simulink model "MATLABPSB_BASED_MODELING_AND_Sim"  (Simulink 8.1)
settings: Solver=FixedStepDiscrete  SolverMode=SingleTasking  StartTime=0.0  StopTime=1  FixedStep=Ts  MaxStep=Ts*2  RelTol=1e-4  AbsTol=1e-4
PreLoadFcn:
  | Ts=50e-6;
values from neighbouring files (symbols this model uses):
  A = 1.5    [LoadSimulation.m]
undefined symbols (not defined in the file or in its folder): DiscIntNeverNeededParam, find_system
libraries: powerlib x205, powerlib_extras x39
(part 1 of 5)
Description:
  | Copyright 2008-2012 The MathWorks, Inc.
settings Model: Creator=MathWorks  LastModifiedBy=LALIT  ExtModeTrigMode=oneshot  ExtModeArmWhenConnect=off  ExtModeAutoUpdateStatusClock=off
settings DataIOCC: LimitDataPoints=off  SaveFinalState=on  SaveFormat=StructureWithTime  SaveOutput=off  SaveTime=off  SignalLoggingName=sigsOut
settings OptimizationCC: BooleanDataType=off  InitFltsAndDblsToZero=on  EfficientMapNaN2IntZero=off
settings DebuggingCC: CheckExecutionContextPreStartOutputMsg=on  CheckExecutionContextRuntimeOutputMsg=on  SignalResolutionControl=TryResolveAllWithWarning  SolverPrmCheckMsg=none  MultiTaskDSMMsg=warning  MultiTaskCondExecSysMsg=none  StrictBusMsg=None
settings HardwareCC: TargetUnknown=on
settings RTWCC: IncludeERTFirstTime=on

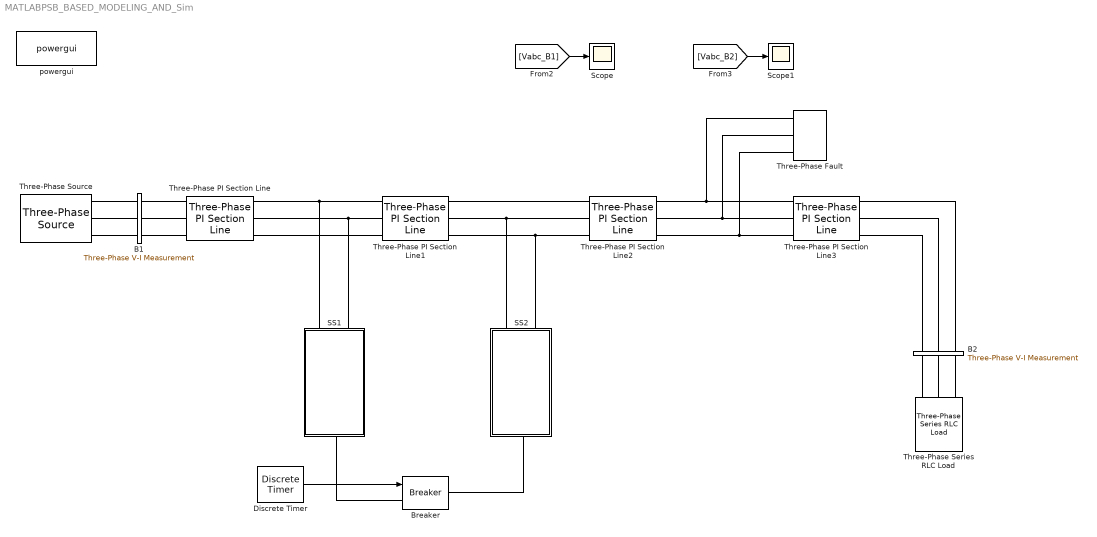
== system MATLABPSB_BASED_MODELING_AND_Sim ==
  B1 : powerlib/Measurements/Three-Phase V-I Measurement  VoltageMeasurement=phase-to-ground  SetLabelV=on  LabelV=Vabc_B1  Vpu=on  VpuLL=off  CurrentMeasurement=yes  SetLabelI=on  LabelI=Iabc_B1  Ipu=off  Pbase=100e6  Vbase=220e3  OutputType=Complex  PhasorSimulation=off  PSBequivalent=0
  B2 : powerlib/Measurements/Three-Phase V-I Measurement  VoltageMeasurement=phase-to-phase  SetLabelV=on  LabelV=Vabc_B2  Vpu=off  VpuLL=on  CurrentMeasurement=yes  SetLabelI=on  LabelI=Iabc_B2  Ipu=off  Pbase=100e6  Vbase=220e3  OutputType=Complex  PhasorSimulation=off  PSBequivalent=0
  Breaker : powerlib/Elements/Breaker  BreakerResistance=0.01  InitialState=0  SnubberResistance=1e6  SnubberCapacitance=inf  SwitchingTimes="[ 1/60  5/60 ]"  External=on  Measurements=None  MoreParameters=off  NoBreakLoop=off
  Discrete Timer : powerlib_extras/Discrete  Control Blocks/Discrete Timer  t=[0 1]  e=[0 1]  Ts=Ts
  SS1 : Subsystem
  SS2 : Subsystem
  Scope : Scope
      settings: SaveName=ScopeData10  Decimation=5
  Scope1 : Scope
      settings: YMin=-1.1  YMax=1.1  Decimation=5
  Three-Phase PI Section Line{,1..3} (4 alike) : powerlib/Elements/Three-Phase PI Section Line  LConnTagsString=a|b|c  RConnTagsString=A|B|C  Frequency=50  Resistances=[ 0.01273 0.3864]  Inductances="[ 0.9337e-3  4.1264e-3]"  Capacitances=[12.74e-9 7.751e-9]  Length=100
  Three-Phase Series RLC Load : powerlib/Elements/Three-Phase Series RLC Load  LConnTagsString=A|B|C  Configuration=Y (grounded)  NominalVoltage=220e3  NominalFrequency=50  ActivePower=100e6  InductivePower=0  CapacitivePower=0  Measurements=None  LoadType=constant Z
  Three-Phase Fault : powerlib/Elements/Three-Phase Fault  FaultA=on  FaultB=on  FaultC=on  FaultResistance=50  GroundFault=on  GroundResistance=0.001  External=off  SwitchStatus=[1]  SwitchTimes=[0.3]  InitialStates=[0 0 1]  SnubberResistance=1e6  SnubberCapacitance=inf  Measurements=None
  Three-Phase Source : powerlib/Electrical Sources/Three-Phase Source  Voltage=220e3  PhaseAngle=0  Frequency=50  InternalConnection=Yg  SpecifyImpedance=on  Resistance=0.8929  Inductance=16.58e-3  ShortCircuitLevel=5000e6  BaseVoltage=220e3  XRratio=7  BusType=swing  Pref=0  Qref=0  Qmin=-inf  Qmax=inf
  powergui : powerlib/powergui  Priority=2  SimulationMode=Discrete  SolverType=Tustin  SampleTime=Ts  frequency=60  SPID=off  DisableSnubberDevices=off  DisableRonSwitches=off  DisableVfSwitches=off  SwTol=0  Interpol=off  DisplayEquations=off  frequencyindice=50  Pbase=100e6  ErrMax=1e-4  Iterations=50  UnitsV=kV  UnitsW=MW  FunctionMessages=off  echomessages=off  HookPort=off  EnableUseOfTLC=off  x0status=blocks  RestoreLinks=warning  ResistiveCurrentMeasurement=off  Frange=[0:2:500]  Ylog=off  Xlog=on  ShowGrid=off  save=off  variable=ZData  structure=Va  ZoomFFT=off  StartTime=0.7  cycles=1  DisplayStyle=1  fundamental=60  FreqAxis=off  MaxFrequency=1000  frequencyindicesteady=1  RmsSteady=2  display=off  Ts=0  methode=off
  wires:
  [Vabc_B1] -> Scope/1
  [Vabc_B2] -> Scope1/1
  Discrete Timer/1 -> Breaker/1
  connections:
  SS1/LConn1 -- Three-Phase PI Section Line/RConn1 -- Three-Phase PI Section Line1/LConn1
  Three-Phase Fault/LConn1 -- Three-Phase PI Section Line2/RConn1 -- Three-Phase PI Section Line3/LConn1
  SS1/LConn2 -- Three-Phase PI Section Line/RConn2 -- Three-Phase PI Section Line1/LConn2
  Three-Phase PI Section Line2/LConn2 -- SS2/LConn1 -- Three-Phase PI Section Line1/RConn2
  Three-Phase PI Section Line2/LConn3 -- SS2/LConn2 -- Three-Phase PI Section Line1/RConn3
  Three-Phase Fault/LConn2 -- Three-Phase PI Section Line2/RConn2 -- Three-Phase PI Section Line3/LConn2
  Three-Phase Fault/LConn3 -- Three-Phase PI Section Line2/RConn3 -- Three-Phase PI Section Line3/LConn3
  Three-Phase Source/RConn1 -- B1/LConn1
  Three-Phase PI Section Line1/RConn1 -- Three-Phase PI Section Line2/LConn1
  B1/RConn3 -- Three-Phase PI Section Line/LConn3
  Three-Phase Source/RConn3 -- B1/LConn3
  Three-Phase PI Section Line3/RConn1 -- B2/LConn3
  Three-Phase Source/RConn2 -- B1/LConn2
  B1/RConn1 -- Three-Phase PI Section Line/LConn1
  B1/RConn2 -- Three-Phase PI Section Line/LConn2
  B2/RConn1 -- Three-Phase Series RLC Load/LConn1
  Breaker/LConn1 -- SS1/RConn1
  Breaker/RConn1 -- SS2/RConn1
  B2/RConn2 -- Three-Phase Series RLC Load/LConn2
  Three-Phase PI Section Line3/RConn3 -- B2/LConn1
  Three-Phase PI Section Line/RConn3 -- Three-Phase PI Section Line1/LConn3
  Three-Phase PI Section Line3/RConn2 -- B2/LConn2
  B2/RConn3 -- Three-Phase Series RLC Load/LConn3

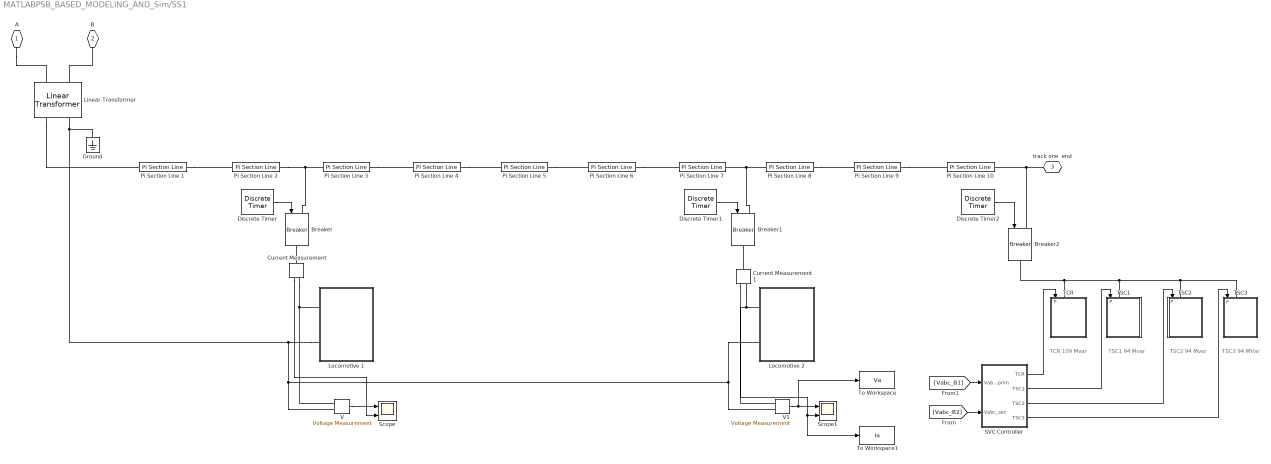
== system MATLABPSB_BASED_MODELING_AND_Sim/SS1 ==
  note: TSC1
      | 94 Mvar
  note: TCR
      | 109 Mvar
  note: TSC2
      | 94 Mvar
  note: TSC3
      | 94 MVar
  Breaker : powerlib/Elements/Breaker  BreakerResistance=0.01  InitialState=0  SnubberResistance=1e6  SnubberCapacitance=inf  SwitchingTimes="[ 1/60  5/60 ]"  External=on  Measurements=None  MoreParameters=off  NoBreakLoop=off
  Breaker1 : powerlib/Elements/Breaker  BreakerResistance=0.01  InitialState=0  SnubberResistance=1e6  SnubberCapacitance=inf  SwitchingTimes="[ 1/60  5/60 ]"  External=on  Measurements=None  MoreParameters=off  NoBreakLoop=off
  Breaker2 : powerlib/Elements/Breaker  BreakerResistance=0.01  InitialState=0  SnubberResistance=1e6  SnubberCapacitance=inf  SwitchingTimes="[ 1/60  5/60 ]"  External=on  Measurements=None  MoreParameters=off  NoBreakLoop=off
  Current Measurement : powerlib/Measurements/Current Measurement  PhasorSimulation=off  OutputType=Complex  PSBequivalent=0
  Current Measurement1 : powerlib/Measurements/Current Measurement  PhasorSimulation=off  OutputType=Complex  PSBequivalent=0
  Discrete Timer : powerlib_extras/Discrete  Control Blocks/Discrete Timer  t=[0 0.01]  e=[0 1]  Ts=Ts
  Discrete Timer1 : powerlib_extras/Discrete  Control Blocks/Discrete Timer  t=[0 0.1]  e=[0 1]  Ts=Ts
  Discrete Timer2 : powerlib_extras/Discrete  Control Blocks/Discrete Timer  t=[0 0.6]  e=[0 1]  Ts=Ts
  Ground : powerlib/Elements/Ground  LConnTagsString=a
  Linear Transformer : powerlib/Elements/Linear Transformer  LConnTagsString=a|b  RConnTagsString=A|B  UNITS=pu  NominalPower=[ 25e6 50 ]  winding1="[ 220e3  0.001  0.06 ]"  winding2="[ 25e3  0.001  0.06 ]"  ThreeWindings=off  winding3=[ 315e3 0.002 0.08 ]  RmLm=[ 500 500 ]  Measurements=None  DataType=off
  Locomotive 1 : Subsystem
  Locomotive 2 : Subsystem
  Pi Section Line {1..10} (10 alike) : powerlib/Elements/Pi Section Line  LConnTagsString=__new0  RConnTagsString=__new0  Frequency=50  Resistance=0.169  Inductance=0.432/(2*pi*50)  Capacitance=0.011e-6  Length=4  PiSections=1  Measurements=None
      settings: AttributesFormatString=\n
  SVC Controller : Subsystem  mask(SVC Controller){OpMode=Voltage regulation, Vref=1.0, KpKi=[0 800], Xs=0.01, Bmin_max=[-1.04  3.23], Bref=0, Ts=Ts}
      mask prompts: OpMode "Operation mode"; Vref "Reference voltage (pu):"; KpKi "Regulator gains [ Kp  Ki ]:"; Xs "Droop (pu/100MVA):"; Bmin_max "Min. and max. primary susceptances [ Bind Bcap] (pu/100MVA):"; Bref "Susceptance Bref (pu/100MVA) (Var control mode):"; Ts "Sample time (s):"
      mask help:
      | This block implements a controller for a Static Var Compensator (SVC) consisting of one thyristor-controlled reactor bank (TCR) and three thyristor-switched capacitor banks (TSCs). Outputs TCR, TSC1, TSC2 and TSC3 are vectors of six pulses for the TCR and the three TSCs.
      | In Voltage control mode the primary voltage (Vabc_prim) is controlled at Vref within the maximum inductive and capacitive susceptance range and droop setting. In Var control mode the SVC susceptance  is  kept constant at Bref (Bref<0 for inductive mode).
      | Thyristor pulses are synchronized on secondary line-to-line voltages (Vabc_sec) of the coupling transformer, assuming a Wye/Delta (D1) connection.
      mask init:
      | Kp=KpKi(1);
      | Ki=KpKi(2);
      | Bmin=Bmin_max(1);
      | Bmax=Bmin_max(2);
      mask TypeOptions OpMode: Voltage regulation | Var control (Fixed susceptance Bref)
  Scope : Scope  NumInputPorts=2
      settings: YMin=-40000~-5  YMax=40000~5  SaveName=ScopeData8  Decimation=5
  Scope1 : Scope  NumInputPorts=2
      settings: YMin=-40000~-5  YMax=40000~5  SaveName=ScopeData9  Decimation=5
  TCR : Subsystem  LoadFcn=find_system(gcs,'FollowLinks', 'on', 'LookUnderMasks', 'all');  mask(TCR branch){Ltcr=18.7e-3, Q=50, ParS=[500 250e-9], ParT=[1e-3  1*15]}
      mask prompts: Ltcr "TCR Inductance (H) :"; Q "Quality factor:"; ParS "Thyristor snubber: [ R (ohm)   C (F)  ]"; ParT "Thyristor data: [ Ron (ohm)   Vf (volt) ]"
      mask init:
      | Rtcr=(2*pi*60) * Ltcr / Q;
      | Rsnub=ParS(1);
      | Csnub=ParS(2);
      | Ron=ParT(1);
      | Vf=ParT(2);
      mask Display:
      | plot(0,0);plot(125,220)
      | plot([62 62 37 37 49 25 37],[15 39 39 58 76 76 58])
      | plot([62 87 87 99 87 75 87],[39 39 58 58 76 58 58])
      | plot([25 49],[58 58]);plot([37 25],[58 49])
      | plot([75 99],[76 76]);plot([87 99],[76 85])
      | plot([37 37 87 87],[76 95 95 76])
      | plot([62 62],[95 122]);plot([62 62],[164 186])
      | plot([62 72 78 79 78 72 62],[122 123 125 129 133 135 136])
      | plot([62 72 78 79 78 72 62],14+[122 123 125 129 133 135 136])
      | plot([62 72 78 79 78 72 62],28+[122 123 125 129 133 135 136])
  TSC1 : Subsystem  mask(TSC branch){Ccmt=308.4e-6, ParL=[1.13e-3 4.26e-3*2 191.7/2], ParS=[500 250e-9], ParT=[1e-3  1*15]}
      mask prompts: Ccmt "Capacitance (F) :"; ParL "[ Inductance (H)  Rseries (ohm)  Rparallel (ohm)  ]"; ParS "Thyristor snubber: [ R (ohm)   C (F)  ]"; ParT "Thyristor data: [ Ron (ohm)  Vf (volt) ]"
      mask init:
      | Lcmt=ParL(1);
      | Rseries=ParL(2);
      | Rparallel=ParL(3);
      | Rsnub=ParS(1);
      | Csnub=ParS(2);
      | Ron=ParT(1);
      | Vf=ParT(2);
      mask Display:
      | plot(0,0);plot(125,220)
      | plot([62 62 37 37 49 25 37],[15 39 39 58 76 76 58])
      | plot([62 87 87 99 87 75 87],[39 39 58 58 76 58 58])
      | plot([25 49],[58 58]);plot([37 25],[58 49])
      | plot([75 99],[76 76]);plot([87 99],[76 85])
      | plot([37 37 87 87],[76 95 95 76])
      | plot([62 62],[95 133]);plot([62 62],[164 183])
      | plot([62 69 73 78 81 82],13+[120 120 119 118 117 115])
      | plot([62 55 51 46 43 42],13+[120 120 119 118 117 115])
      | plot([42 82],[145 145])
      | plot([62 62],[145 164])
  TSC2 : Subsystem  mask(TSC branch){Ccmt=308.4e-6, ParL=[1.13e-3 4.26e-3*2 191.7/2], ParS=[500 250e-9], ParT=[1e-3 1*15]}
      mask prompts: Ccmt "Capacitance (F) :"; ParL "[ Inductance (H)  Rseries (ohm)  Rparallel (ohm)  ]"; ParS "Thyristor snubber: [ R (ohm)   C (F)  ]"; ParT "Thyristor data: [ Ron (ohm)  Vf (volt) ]"
      mask init:
      | Lcmt=ParL(1);
      | Rseries=ParL(2);
      | Rparallel=ParL(3);
      | Rsnub=ParS(1);
      | Csnub=ParS(2);
      | Ron=ParT(1);
      | Vf=ParT(2);
      mask Display:
      | plot(0,0);plot(125,220)
      | plot([62 62 37 37 49 25 37],[15 39 39 58 76 76 58])
      | plot([62 87 87 99 87 75 87],[39 39 58 58 76 58 58])
      | plot([25 49],[58 58]);plot([37 25],[58 49])
      | plot([75 99],[76 76]);plot([87 99],[76 85])
      | plot([37 37 87 87],[76 95 95 76])
      | plot([62 62],[95 133]);plot([62 62],[164 183])
      | plot([62 69 73 78 81 82],13+[120 120 119 118 117 115])
      | plot([62 55 51 46 43 42],13+[120 120 119 118 117 115])
      | plot([42 82],[145 145])
      | plot([62 62],[145 164])
  TSC3 : Subsystem  mask(TSC branch){Ccmt=308.4e-6, ParL=[1.13e-3 4.26e-3*2 191.7/2], ParS=[500 250e-9], ParT=[1e-3 1*15]}
      mask prompts: Ccmt "Capacitance (F) :"; ParL "[ Inductance (H)  Rseries (ohm)  Rparallel (ohm)  ]"; ParS "Thyristor snubber: [ R (ohm)   C (F)  ]"; ParT "Thyristor data: [ Ron (ohm)  Vf (volt) ]"
      mask init:
      | Lcmt=ParL(1);
      | Rseries=ParL(2);
      | Rparallel=ParL(3);
      | Rsnub=ParS(1);
      | Csnub=ParS(2);
      | Ron=ParT(1);
      | Vf=ParT(2);
      mask Display:
      | plot(0,0);plot(125,220)
      | plot([62 62 37 37 49 25 37],[15 39 39 58 76 76 58])
      | plot([62 87 87 99 87 75 87],[39 39 58 58 76 58 58])
      | plot([25 49],[58 58]);plot([37 25],[58 49])
      | plot([75 99],[76 76]);plot([87 99],[76 85])
      | plot([37 37 87 87],[76 95 95 76])
      | plot([62 62],[95 133]);plot([62 62],[164 183])
      | plot([62 69 73 78 81 82],13+[120 120 119 118 117 115])
      | plot([62 55 51 46 43 42],13+[120 120 119 118 117 115])
      | plot([42 82],[145 145])
      | plot([62 62],[145 164])
  To Workspace : ToWorkspace  VariableName=Va  SampleTime=-1  SaveFormat=Structure With Time
  To Workspace1 : ToWorkspace  VariableName=Ia  SampleTime=-1  SaveFormat=Structure With Time
  V : powerlib/Measurements/Voltage Measurement  PhasorSimulation=off  OutputType=Complex  PSBequivalent=0
  V1 : powerlib/Measurements/Voltage Measurement  PhasorSimulation=off  OutputType=Complex  PSBequivalent=0
  A : PMIOPort  Tag=PMCPort  Port=1  Side=Left
  B : PMIOPort  Tag=PMCPort  Port=2  Side=Left
  track one  end : PMIOPort  Tag=PMCPort  Port=3  Side=Right
  wires:
  V/1 -> Scope/1
  Discrete Timer/1 -> Breaker/1
  V1/1 -> Scope1/1, To Workspace/1
  Discrete Timer1/1 -> Breaker1/1
  Discrete Timer2/1 -> Breaker2/1
  Current Measurement/1 -> Scope/2
  Current Measurement1/1 -> Scope1/2, To Workspace1/1
  [Vabc_B2] -> SVC Controller/2(Vabc_sec)
  [Vabc_B1] -> SVC Controller/1(Vabc_prim)
  SVC Controller/1(TCR) -> TCR/1(P)
  SVC Controller/2(TSC1) -> TSC1/1(P)
  SVC Controller/3(TSC2) -> TSC2/1(P)
  SVC Controller/4(TSC3) -> TSC3/1(P)
  connections:
  A/RConn1 -- Linear Transformer/LConn1
  Linear Transformer/LConn2 -- B/RConn1
  Locomotive 1/LConn2 -- Linear Transformer/RConn2 -- Ground/LConn1 -- Locomotive 2/LConn2 -- V1/LConn2 -- V/LConn2
  Linear Transformer/RConn1 -- Pi Section Line 1/LConn1
  Pi Section Line 1/RConn1 -- Pi Section Line 2/LConn1
  V/LConn1 -- Locomotive 1/LConn1 -- Current Measurement/RConn1
  Pi Section Line 3/RConn1 -- Pi Section Line 4/LConn1
  Pi Section Line 4/RConn1 -- Pi Section Line 5/LConn1
  Pi Section Line 5/RConn1 -- Pi Section Line 6/LConn1
  Pi Section Line 6/RConn1 -- Pi Section Line 7/LConn1
  Pi Section Line 8/LConn1 -- Pi Section Line 7/RConn1 -- Breaker1/LConn1
  Pi Section Line 8/RConn1 -- Pi Section Line 9/LConn1
  Pi Section Line 9/RConn1 -- Pi Section Line 10/LConn1
  track one  end/RConn1 -- Pi Section Line 10/RConn1 -- Breaker2/LConn1
  Pi Section Line 2/RConn1 -- Pi Section Line 3/LConn1 -- Breaker/LConn1
  V1/LConn1 -- Locomotive 2/LConn1 -- Current Measurement1/RConn1
  Current Measurement/LConn1 -- Breaker/RConn1
  Current Measurement1/LConn1 -- Breaker1/RConn1
  TCR/LConn1 -- Breaker2/RConn1 -- TSC1/LConn1 -- TSC2/LConn1 -- TSC3/LConn1

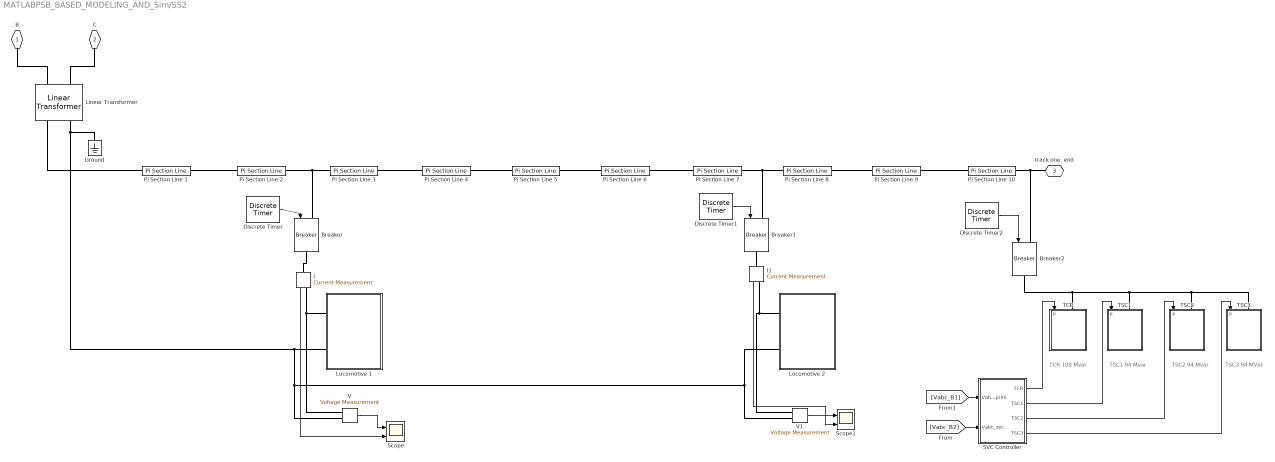
== system MATLABPSB_BASED_MODELING_AND_Sim/SS2 ==
  note: TSC3
      | 94 MVar
  note: TSC2
      | 94 Mvar
  note: TCR
      | 109 Mvar
  note: TSC1
      | 94 Mvar
  Breaker : powerlib/Elements/Breaker  BreakerResistance=0.01  InitialState=0  SnubberResistance=1e6  SnubberCapacitance=inf  SwitchingTimes="[ 1/60  5/60 ]"  External=on  Measurements=None  MoreParameters=off  NoBreakLoop=off
  Breaker1 : powerlib/Elements/Breaker  BreakerResistance=0.01  InitialState=0  SnubberResistance=1e6  SnubberCapacitance=inf  SwitchingTimes="[ 1/60  5/60 ]"  External=on  Measurements=None  MoreParameters=off  NoBreakLoop=off
  Breaker2 : powerlib/Elements/Breaker  BreakerResistance=0.01  InitialState=0  SnubberResistance=1e6  SnubberCapacitance=inf  SwitchingTimes="[ 1/60  5/60 ]"  External=on  Measurements=None  MoreParameters=off  NoBreakLoop=off
  Discrete Timer : powerlib_extras/Discrete  Control Blocks/Discrete Timer  t=[0 0.01]  e=[0 1]  Ts=Ts
  Discrete Timer1 : powerlib_extras/Discrete  Control Blocks/Discrete Timer  t=[0 0.1]  e=[0 1]  Ts=Ts
  Discrete Timer2 : powerlib_extras/Discrete  Control Blocks/Discrete Timer  t=[0 0.6]  e=[0 1]  Ts=Ts
  Ground : powerlib/Elements/Ground  LConnTagsString=a
  I : powerlib/Measurements/Current Measurement  PhasorSimulation=off  OutputType=Complex  PSBequivalent=0
  I1 : powerlib/Measurements/Current Measurement  PhasorSimulation=off  OutputType=Complex  PSBequivalent=0
  Linear Transformer : powerlib/Elements/Linear Transformer  LConnTagsString=a|b  RConnTagsString=A|B  UNITS=pu  NominalPower=[ 25e6 50 ]  winding1="[ 220e3  0.001  0.06 ]"  winding2="[ 25e3  0.001  0.06 ]"  ThreeWindings=off  winding3=[ 315e3 0.002 0.08 ]  RmLm=[ 500 500 ]  Measurements=None  DataType=off
  Locomotive 1 : Subsystem
  Locomotive 2 : Subsystem
  Pi Section Line {1..10} (10 alike) : powerlib/Elements/Pi Section Line  LConnTagsString=__new0  RConnTagsString=__new0  Frequency=50  Resistance=0.169  Inductance=0.432/(2*pi*50)  Capacitance=0.011e-6  Length=4  PiSections=1  Measurements=None
      settings: AttributesFormatString=\n
  SVC Controller : Subsystem  mask(SVC Controller){OpMode=Voltage regulation, Vref=1.0, KpKi=[0 800], Xs=0.01, Bmin_max=[-1.04  3.23], Bref=0, Ts=Ts}
      mask prompts: OpMode "Operation mode"; Vref "Reference voltage (pu):"; KpKi "Regulator gains [ Kp  Ki ]:"; Xs "Droop (pu/100MVA):"; Bmin_max "Min. and max. primary susceptances [ Bind Bcap] (pu/100MVA):"; Bref "Susceptance Bref (pu/100MVA) (Var control mode):"; Ts "Sample time (s):"
      mask help:
      | This block implements a controller for a Static Var Compensator (SVC) consisting of one thyristor-controlled reactor bank (TCR) and three thyristor-switched capacitor banks (TSCs). Outputs TCR, TSC1, TSC2 and TSC3 are vectors of six pulses for the TCR and the three TSCs.
      | In Voltage control mode the primary voltage (Vabc_prim) is controlled at Vref within the maximum inductive and capacitive susceptance range and droop setting. In Var control mode the SVC susceptance  is  kept constant at Bref (Bref<0 for inductive mode).
      | Thyristor pulses are synchronized on secondary line-to-line voltages (Vabc_sec) of the coupling transformer, assuming a Wye/Delta (D1) connection.
      mask init:
      | Kp=KpKi(1);
      | Ki=KpKi(2);
      | Bmin=Bmin_max(1);
      | Bmax=Bmin_max(2);
      mask TypeOptions OpMode: Voltage regulation | Var control (Fixed susceptance Bref)
  Scope : Scope  NumInputPorts=2
      settings: YMin=-40000~-5  YMax=40000~5  SaveName=ScopeData2  Decimation=5
  Scope1 : Scope  NumInputPorts=2
      settings: YMin=-60000~-5  YMax=60000~5  SaveName=ScopeData7  Decimation=5
  TCR : Subsystem  LoadFcn=find_system(gcs,'FollowLinks', 'on', 'LookUnderMasks', 'all');  mask(TCR branch){Ltcr=18.7e-3, Q=50, ParS=[500 250e-9], ParT=[1e-3  1*15]}
      mask prompts: Ltcr "TCR Inductance (H) :"; Q "Quality factor:"; ParS "Thyristor snubber: [ R (ohm)   C (F)  ]"; ParT "Thyristor data: [ Ron (ohm)   Vf (volt) ]"
      mask init:
      | Rtcr=(2*pi*60) * Ltcr / Q;
      | Rsnub=ParS(1);
      | Csnub=ParS(2);
      | Ron=ParT(1);
      | Vf=ParT(2);
      mask Display:
      | plot(0,0);plot(125,220)
      | plot([62 62 37 37 49 25 37],[15 39 39 58 76 76 58])
      | plot([62 87 87 99 87 75 87],[39 39 58 58 76 58 58])
      | plot([25 49],[58 58]);plot([37 25],[58 49])
      | plot([75 99],[76 76]);plot([87 99],[76 85])
      | plot([37 37 87 87],[76 95 95 76])
      | plot([62 62],[95 122]);plot([62 62],[164 186])
      | plot([62 72 78 79 78 72 62],[122 123 125 129 133 135 136])
      | plot([62 72 78 79 78 72 62],14+[122 123 125 129 133 135 136])
      | plot([62 72 78 79 78 72 62],28+[122 123 125 129 133 135 136])
  TSC1 : Subsystem  mask(TSC branch){Ccmt=308.4e-6, ParL=[1.13e-3 4.26e-3*2 191.7/2], ParS=[500 250e-9], ParT=[1e-3  1*15]}
      mask prompts: Ccmt "Capacitance (F) :"; ParL "[ Inductance (H)  Rseries (ohm)  Rparallel (ohm)  ]"; ParS "Thyristor snubber: [ R (ohm)   C (F)  ]"; ParT "Thyristor data: [ Ron (ohm)  Vf (volt) ]"
      mask init:
      | Lcmt=ParL(1);
      | Rseries=ParL(2);
      | Rparallel=ParL(3);
      | Rsnub=ParS(1);
      | Csnub=ParS(2);
      | Ron=ParT(1);
      | Vf=ParT(2);
      mask Display:
      | plot(0,0);plot(125,220)
      | plot([62 62 37 37 49 25 37],[15 39 39 58 76 76 58])
      | plot([62 87 87 99 87 75 87],[39 39 58 58 76 58 58])
      | plot([25 49],[58 58]);plot([37 25],[58 49])
      | plot([75 99],[76 76]);plot([87 99],[76 85])
      | plot([37 37 87 87],[76 95 95 76])
      | plot([62 62],[95 133]);plot([62 62],[164 183])
      | plot([62 69 73 78 81 82],13+[120 120 119 118 117 115])
      | plot([62 55 51 46 43 42],13+[120 120 119 118 117 115])
      | plot([42 82],[145 145])
      | plot([62 62],[145 164])
  TSC2 : Subsystem  mask(TSC branch){Ccmt=308.4e-6, ParL=[1.13e-3 4.26e-3*2 191.7/2], ParS=[500 250e-9], ParT=[1e-3 1*15]}
      mask prompts: Ccmt "Capacitance (F) :"; ParL "[ Inductance (H)  Rseries (ohm)  Rparallel (ohm)  ]"; ParS "Thyristor snubber: [ R (ohm)   C (F)  ]"; ParT "Thyristor data: [ Ron (ohm)  Vf (volt) ]"
      mask init:
      | Lcmt=ParL(1);
      | Rseries=ParL(2);
      | Rparallel=ParL(3);
      | Rsnub=ParS(1);
      | Csnub=ParS(2);
      | Ron=ParT(1);
      | Vf=ParT(2);
      mask Display:
      | plot(0,0);plot(125,220)
      | plot([62 62 37 37 49 25 37],[15 39 39 58 76 76 58])
      | plot([62 87 87 99 87 75 87],[39 39 58 58 76 58 58])
      | plot([25 49],[58 58]);plot([37 25],[58 49])
      | plot([75 99],[76 76]);plot([87 99],[76 85])
      | plot([37 37 87 87],[76 95 95 76])
      | plot([62 62],[95 133]);plot([62 62],[164 183])
      | plot([62 69 73 78 81 82],13+[120 120 119 118 117 115])
      | plot([62 55 51 46 43 42],13+[120 120 119 118 117 115])
      | plot([42 82],[145 145])
      | plot([62 62],[145 164])
  TSC3 : Subsystem  mask(TSC branch){Ccmt=308.4e-6, ParL=[1.13e-3 4.26e-3*2 191.7/2], ParS=[500 250e-9], ParT=[1e-3 1*15]}
      mask prompts: Ccmt "Capacitance (F) :"; ParL "[ Inductance (H)  Rseries (ohm)  Rparallel (ohm)  ]"; ParS "Thyristor snubber: [ R (ohm)   C (F)  ]"; ParT "Thyristor data: [ Ron (ohm)  Vf (volt) ]"
      mask init:
      | Lcmt=ParL(1);
      | Rseries=ParL(2);
      | Rparallel=ParL(3);
      | Rsnub=ParS(1);
      | Csnub=ParS(2);
      | Ron=ParT(1);
      | Vf=ParT(2);
      mask Display:
      | plot(0,0);plot(125,220)
      | plot([62 62 37 37 49 25 37],[15 39 39 58 76 76 58])
      | plot([62 87 87 99 87 75 87],[39 39 58 58 76 58 58])
      | plot([25 49],[58 58]);plot([37 25],[58 49])
      | plot([75 99],[76 76]);plot([87 99],[76 85])
      | plot([37 37 87 87],[76 95 95 76])
      | plot([62 62],[95 133]);plot([62 62],[164 183])
      | plot([62 69 73 78 81 82],13+[120 120 119 118 117 115])
      | plot([62 55 51 46 43 42],13+[120 120 119 118 117 115])
      | plot([42 82],[145 145])
      | plot([62 62],[145 164])
  V : powerlib/Measurements/Voltage Measurement  PhasorSimulation=off  OutputType=Complex  PSBequivalent=0
  V1 : powerlib/Measurements/Voltage Measurement  PhasorSimulation=off  OutputType=Complex  PSBequivalent=0
  B : PMIOPort  Tag=PMCPort  Port=1  Side=Left
  C : PMIOPort  Tag=PMCPort  Port=2  Side=Left
  track one  end : PMIOPort  Tag=PMCPort  Port=3  Side=Right
  wires:
  V/1 -> Scope/1
  Discrete Timer/1 -> Breaker/1
  V1/1 -> Scope1/1
  Discrete Timer1/1 -> Breaker1/1
  Discrete Timer2/1 -> Breaker2/1
  I/1 -> Scope/2
  I1/1 -> Scope1/2
  [Vabc_B2] -> SVC Controller/2(Vabc_sec)
  [Vabc_B1] -> SVC Controller/1(Vabc_prim)
  SVC Controller/1(TCR) -> TCR/1(P)
  SVC Controller/2(TSC1) -> TSC1/1(P)
  SVC Controller/3(TSC2) -> TSC2/1(P)
  SVC Controller/4(TSC3) -> TSC3/1(P)
  connections:
  B/RConn1 -- Linear Transformer/LConn1
  Linear Transformer/LConn2 -- C/RConn1
  Linear Transformer/RConn1 -- Pi Section Line 1/LConn1
  Pi Section Line 1/RConn1 -- Pi Section Line 2/LConn1
  V/LConn1 -- I/RConn1 -- Locomotive 1/LConn1
  Pi Section Line 3/RConn1 -- Pi Section Line 4/LConn1
  Pi Section Line 4/RConn1 -- Pi Section Line 5/LConn1
  Pi Section Line 5/RConn1 -- Pi Section Line 6/LConn1
  Pi Section Line 6/RConn1 -- Pi Section Line 7/LConn1
  Pi Section Line 8/LConn1 -- Pi Section Line 7/RConn1 -- Breaker1/LConn1
  Pi Section Line 8/RConn1 -- Pi Section Line 9/LConn1
  Pi Section Line 9/RConn1 -- Pi Section Line 10/LConn1
  track one  end/RConn1 -- Pi Section Line 10/RConn1 -- Breaker2/LConn1
  Pi Section Line 2/RConn1 -- Pi Section Line 3/LConn1 -- Breaker/LConn1
  Locomotive 2/LConn1 -- V1/LConn1 -- I1/RConn1
  Locomotive 2/LConn2 -- V1/LConn2 -- Locomotive 1/LConn2 -- Linear Transformer/RConn2 -- Ground/LConn1 -- V/LConn2
  I/LConn1 -- Breaker/RConn1
  I1/LConn1 -- Breaker1/RConn1
  TSC1/LConn2 -- TSC2/LConn2 -- TSC3/LConn2 -- TCR/LConn2 -- Breaker2/RConn1

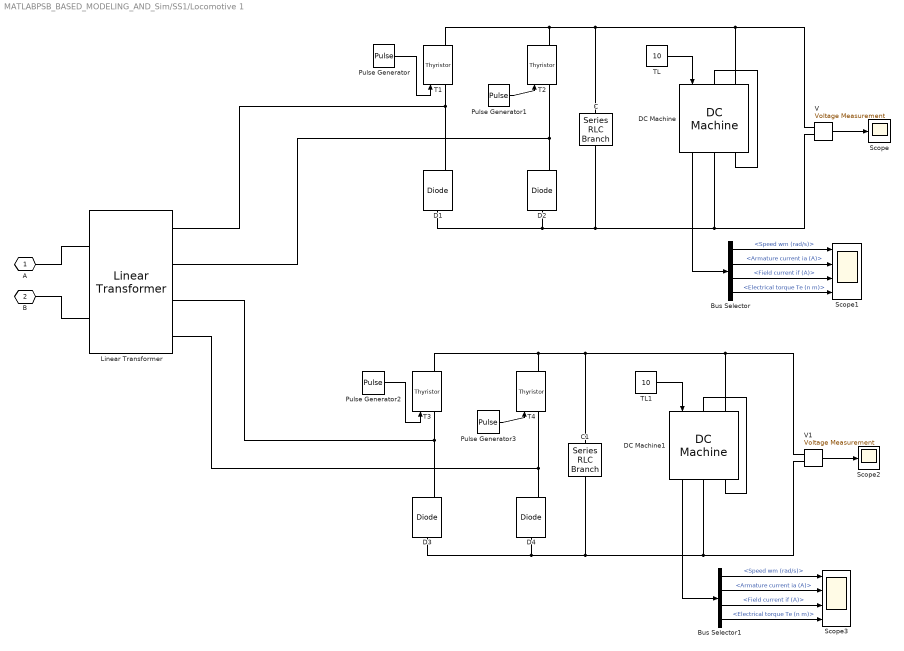
== system MATLABPSB_BASED_MODELING_AND_Sim/SS1/Locomotive 1 ==
  Bus Selector : BusSelector  OutputSignals=Speed wm (rad/s),Armature current ia (A),Field current if (A),Electrical torque Te (n m)
  Bus Selector1 : BusSelector  OutputSignals=Speed wm (rad/s),Armature current ia (A),Field current if (A),Electrical torque Te (n m)
  C : powerlib/Elements/Series RLC Branch  LConnTagsString=__new0  RConnTagsString=__new0  BranchType=C  Resistance=1000  Inductance=1e-3  SetiL0=off  InitialCurrent=0  Capacitance=2000e-6  Setx0=on  InitialVoltage=400  Measurements=None
  C1 : powerlib/Elements/Series RLC Branch  LConnTagsString=__new0  RConnTagsString=__new0  BranchType=C  Resistance=1000  Inductance=1e-3  SetiL0=off  InitialCurrent=0  Capacitance=2000e-6  Setx0=on  InitialVoltage=400  Measurements=None
  D{1..4} (4 alike) : powerlib/Power Electronics/Diode  Ron=0.001  Lon=0  Vf=0.8  IC=0  UseSnubber=off  Rs=500  Cs=250e-9  Measurements=on
  DC Machine : powerlib/Machines/DC Machine  PresetModel=No  MechanicalLoad=Torque TL  FieldType=Wound  ShowDetailedParameters=on  RLa="[ 2.6  150e-3]"  RLf=[0.6 20e-3]  Laf=1.8  MachineConstant=Torque constant (N.m/A)  Ke=1.8  Kt=1.8  J=0.1  Bm=0  Tf=0  w0=1  Ifinit=1  TsPowergui=0  TsBlock=-1
  DC Machine1 : powerlib/Machines/DC Machine  PresetModel=No  MechanicalLoad=Torque TL  FieldType=Wound  ShowDetailedParameters=on  RLa="[ 2.6  150e-3]"  RLf=[0.6 20e-3]  Laf=1.8  MachineConstant=Torque constant (N.m/A)  Ke=1.8  Kt=1.8  J=0.1  Bm=0  Tf=0  w0=1  Ifinit=1  TsPowergui=0  TsBlock=-1
  Linear Transformer : powerlib/Elements/Linear Transformer  LConnTagsString=a|b  RConnTagsString=A|B|C|D  UNITS=pu  NominalPower=[ 10e6 50 ]  winding1="[ 25e3  0.0001  0.04 ]"  winding2="[ 400  0.0001  0.02 ]"  ThreeWindings=on  winding3="[ 400  0.0001  0.02 ]"  RmLm=[ 500 500 ]  Measurements=None  DataType=off
  Pulse Generator : DiscretePulseGenerator  PulseType=Time based  Period=20e-3  PulseWidth=3
  Pulse Generator1 : DiscretePulseGenerator  PulseType=Time based  Period=20e-3  PulseWidth=3  PhaseDelay=10e-3
  Pulse Generator2 : DiscretePulseGenerator  PulseType=Time based  Period=20e-3  PulseWidth=3
  Pulse Generator3 : DiscretePulseGenerator  PulseType=Time based  Period=20e-3  PulseWidth=3  PhaseDelay=10e-3
  Scope : Scope
      settings: YMin=-50  YMax=800  SaveName=ScopeData3  Decimation=5
  Scope1 : Scope  NumInputPorts=4
      settings: YMin=0~-5~-5~-5  YMax=100~5~5~20  SaveName=ScopeData4  Decimation=5
  Scope2 : Scope
      settings: YMin=-50  YMax=800  SaveName=ScopeData5  Decimation=5
  Scope3 : Scope  NumInputPorts=4
      settings: YMin=0~-5~-5~-5  YMax=100~5~5~20  SaveName=ScopeData6  Decimation=5
  T{1..4} (4 alike) : powerlib/Power Electronics/Thyristor  Ron=0.001  Lon=0  Vf=0.8  IC=0  Rs=500  Cs=250e-9  Measurements=on
  TL : Constant  Value=10
  TL1 : Constant  Value=10
  V : powerlib/Measurements/Voltage Measurement  PhasorSimulation=off  OutputType=Complex  PSBequivalent=0
  V1 : powerlib/Measurements/Voltage Measurement  PhasorSimulation=off  OutputType=Complex  PSBequivalent=0
  A : PMIOPort  Tag=PMCPort  Port=1  Side=Left
  B : PMIOPort  Tag=PMCPort  Port=2  Side=Left
  wires:
  Pulse Generator/1 -> T1/1
  Pulse Generator1/1 -> T2/1
  V/1 -> Scope/1
  TL/1 -> DC Machine/1
  DC Machine/1 -> Bus Selector/1
  Bus Selector/1 -> Scope1/1  "<Speed wm (rad/s)>"
  Bus Selector/2 -> Scope1/2  "<Armature current ia (A)>"
  Bus Selector/3 -> Scope1/3  "<Field current if (A)>"
  Bus Selector/4 -> Scope1/4  "<Electrical torque Te (n m)>"
  Pulse Generator2/1 -> T3/1
  Pulse Generator3/1 -> T4/1
  V1/1 -> Scope2/1
  TL1/1 -> DC Machine1/1
  DC Machine1/1 -> Bus Selector1/1
  Bus Selector1/1 -> Scope3/1  "<Speed wm (rad/s)>"
  Bus Selector1/2 -> Scope3/2  "<Armature current ia (A)>"
  Bus Selector1/3 -> Scope3/3  "<Field current if (A)>"
  Bus Selector1/4 -> Scope3/4  "<Electrical torque Te (n m)>"
  connections:
  Linear Transformer/RConn1 -- T1/LConn1 -- D1/RConn1
  Linear Transformer/RConn2 -- T2/LConn1 -- D2/RConn1
  T1/RConn1 -- T2/RConn1 -- C/LConn1 -- V/LConn1 -- DC Machine/LConn2
  D1/LConn1 -- D2/LConn1 -- C/RConn1 -- V/LConn2 -- DC Machine/RConn1
  DC Machine/RConn2 -- DC Machine/LConn1
  C1/LConn1 -- T3/RConn1 -- T4/RConn1 -- V1/LConn1 -- DC Machine1/LConn2
  C1/RConn1 -- D3/LConn1 -- D4/LConn1 -- V1/LConn2 -- DC Machine1/RConn1
  DC Machine1/RConn2 -- DC Machine1/LConn1
  D4/RConn1 -- T4/LConn1 -- Linear Transformer/RConn4
  D3/RConn1 -- T3/LConn1 -- Linear Transformer/RConn3
  A/RConn1 -- Linear Transformer/LConn1
  B/RConn1 -- Linear Transformer/LConn2

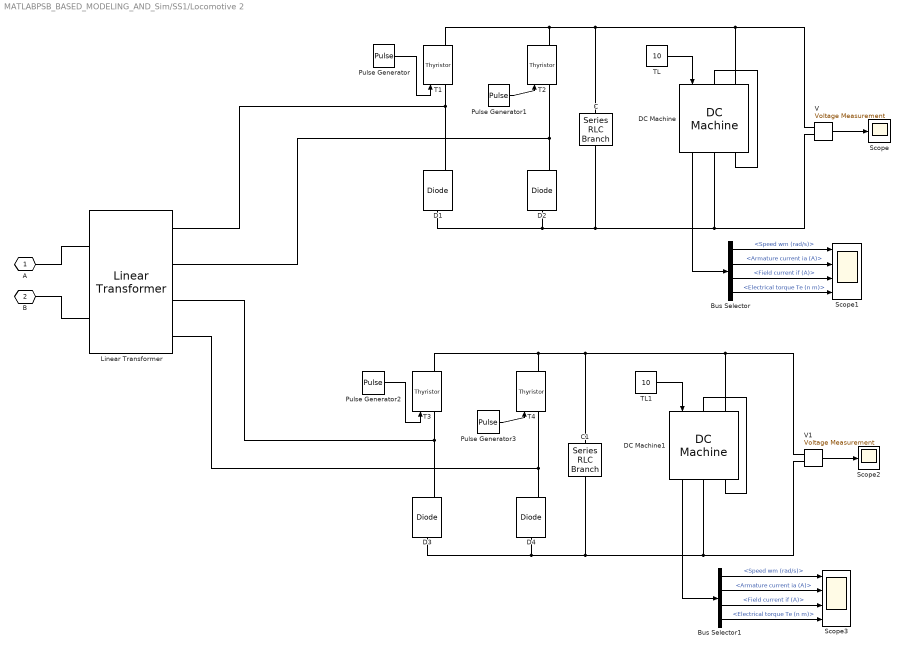
== system MATLABPSB_BASED_MODELING_AND_Sim/SS1/Locomotive 2 ==
  Bus Selector : BusSelector  OutputSignals=Speed wm (rad/s),Armature current ia (A),Field current if (A),Electrical torque Te (n m)
  Bus Selector1 : BusSelector  OutputSignals=Speed wm (rad/s),Armature current ia (A),Field current if (A),Electrical torque Te (n m)
  C : powerlib/Elements/Series RLC Branch  LConnTagsString=__new0  RConnTagsString=__new0  BranchType=C  Resistance=1000  Inductance=1e-3  SetiL0=off  InitialCurrent=0  Capacitance=2000e-6  Setx0=on  InitialVoltage=400  Measurements=None
  C1 : powerlib/Elements/Series RLC Branch  LConnTagsString=__new0  RConnTagsString=__new0  BranchType=C  Resistance=1000  Inductance=1e-3  SetiL0=off  InitialCurrent=0  Capacitance=2000e-6  Setx0=on  InitialVoltage=400  Measurements=None
  D{1..4} (4 alike) : powerlib/Power Electronics/Diode  Ron=0.001  Lon=0  Vf=0.8  IC=0  UseSnubber=off  Rs=500  Cs=250e-9  Measurements=on
  DC Machine : powerlib/Machines/DC Machine  PresetModel=No  MechanicalLoad=Torque TL  FieldType=Wound  ShowDetailedParameters=on  RLa="[ 2.6  150e-3]"  RLf=[0.6 20e-3]  Laf=1.8  MachineConstant=Torque constant (N.m/A)  Ke=1.8  Kt=1.8  J=0.1  Bm=0  Tf=0  w0=1  Ifinit=1  TsPowergui=0  TsBlock=-1
  DC Machine1 : powerlib/Machines/DC Machine  PresetModel=No  MechanicalLoad=Torque TL  FieldType=Wound  ShowDetailedParameters=on  RLa="[ 2.6  150e-3]"  RLf=[0.6 20e-3]  Laf=1.8  MachineConstant=Torque constant (N.m/A)  Ke=1.8  Kt=1.8  J=0.1  Bm=0  Tf=0  w0=1  Ifinit=1  TsPowergui=0  TsBlock=-1
  Linear Transformer : powerlib/Elements/Linear Transformer  LConnTagsString=a|b  RConnTagsString=A|B|C|D  UNITS=pu  NominalPower=[ 10e6 50 ]  winding1="[ 25e3  0.0001  0.04 ]"  winding2="[ 400  0.0001  0.02 ]"  ThreeWindings=on  winding3="[ 400  0.0001  0.02 ]"  RmLm=[ 500 500 ]  Measurements=None  DataType=off
  Pulse Generator : DiscretePulseGenerator  PulseType=Time based  Period=20e-3  PulseWidth=3
  Pulse Generator1 : DiscretePulseGenerator  PulseType=Time based  Period=20e-3  PulseWidth=3  PhaseDelay=10e-3
  Pulse Generator2 : DiscretePulseGenerator  PulseType=Time based  Period=20e-3  PulseWidth=3
  Pulse Generator3 : DiscretePulseGenerator  PulseType=Time based  Period=20e-3  PulseWidth=3  PhaseDelay=10e-3
  Scope : Scope
      settings: YMin=-50  YMax=800  SaveName=ScopeData3  Decimation=5
  Scope1 : Scope  NumInputPorts=4
      settings: YMin=0~-5~-5~-5  YMax=100~5~5~20  SaveName=ScopeData4  Decimation=5
  Scope2 : Scope
      settings: YMin=-50  YMax=800  SaveName=ScopeData5  Decimation=5
  Scope3 : Scope  NumInputPorts=4
      settings: YMin=0~-5~-5~-5  YMax=100~5~5~20  SaveName=ScopeData6  Decimation=5
  T{1..4} (4 alike) : powerlib/Power Electronics/Thyristor  Ron=0.001  Lon=0  Vf=0.8  IC=0  Rs=500  Cs=250e-9  Measurements=on
  TL : Constant  Value=10
  TL1 : Constant  Value=10
  V : powerlib/Measurements/Voltage Measurement  PhasorSimulation=off  OutputType=Complex  PSBequivalent=0
  V1 : powerlib/Measurements/Voltage Measurement  PhasorSimulation=off  OutputType=Complex  PSBequivalent=0
  A : PMIOPort  Tag=PMCPort  Port=1  Side=Left
  B : PMIOPort  Tag=PMCPort  Port=2  Side=Left
  wires:
  Pulse Generator/1 -> T1/1
  Pulse Generator1/1 -> T2/1
  V/1 -> Scope/1
  TL/1 -> DC Machine/1
  DC Machine/1 -> Bus Selector/1
  Bus Selector/1 -> Scope1/1  "<Speed wm (rad/s)>"
  Bus Selector/2 -> Scope1/2  "<Armature current ia (A)>"
  Bus Selector/3 -> Scope1/3  "<Field current if (A)>"
  Bus Selector/4 -> Scope1/4  "<Electrical torque Te (n m)>"
  Pulse Generator2/1 -> T3/1
  Pulse Generator3/1 -> T4/1
  V1/1 -> Scope2/1
  TL1/1 -> DC Machine1/1
  DC Machine1/1 -> Bus Selector1/1
  Bus Selector1/1 -> Scope3/1  "<Speed wm (rad/s)>"
  Bus Selector1/2 -> Scope3/2  "<Armature current ia (A)>"
  Bus Selector1/3 -> Scope3/3  "<Field current if (A)>"
  Bus Selector1/4 -> Scope3/4  "<Electrical torque Te (n m)>"
  connections:
  D1/RConn1 -- Linear Transformer/RConn1 -- T1/LConn1
  D2/RConn1 -- Linear Transformer/RConn2 -- T2/LConn1
  T1/RConn1 -- T2/RConn1 -- C/LConn1 -- V/LConn1 -- DC Machine/LConn2
  D1/LConn1 -- D2/LConn1 -- C/RConn1 -- V/LConn2 -- DC Machine/RConn1
  DC Machine/RConn2 -- DC Machine/LConn1
  T4/RConn1 -- T3/RConn1 -- C1/LConn1 -- V1/LConn1 -- DC Machine1/LConn2
  D4/LConn1 -- D3/LConn1 -- C1/RConn1 -- V1/LConn2 -- DC Machine1/RConn1
  DC Machine1/RConn2 -- DC Machine1/LConn1
  D4/RConn1 -- T4/LConn1 -- Linear Transformer/RConn4
  D3/RConn1 -- T3/LConn1 -- Linear Transformer/RConn3
  A/RConn1 -- Linear Transformer/LConn1
  B/RConn1 -- Linear Transformer/LConn2

== system MATLABPSB_BASED_MODELING_AND_Sim/SS1/SVC Controller ==
  note: Pulses
  note: SVC Controller
  note: Pierre Giroux, Gilbert Sybille
      | Power System Laboratory, IREQ
      | Hydro-Quebec
  note: used for misfiring
      | simulation
  Vabc_prim : Inport  PortDimensions=3
  Vabc_sec : Inport  Port=2  PortDimensions=3
  3-phase signal generator : Subsystem
  Constant : Constant  Value=0.00000001
  Constant1 : Constant  Value=Bref
  Demux : Demux  Outputs=[1 5]
  Distribution Unit : Subsystem  mask(Distribution Unit){ParNom=[333e6 60], Xf_xfo=0.15, Vsec_svc=16e3, L_TCR=18.7e-3, C_TSC=308.4e-6, L_TSC=1.13e-3, hyst_svc=0.1, Ts=Ts}
      mask prompts: ParNom "Transformer nominal power and frequency: [  P (VA)    Freq (Hz)  ]"; Xf_xfo "Transformer total leakage (pu/Pnom):"; Vsec_svc "Nominal secondary voltage (Volts rms ph-ph):"; L_TCR "TCR branch inductance (H):"; C_TSC "TSC branch capacitance (F):"; L_TSC "TSC branch inductance (H)"; hyst_svc "Hysteresis - Distribution unit (pu/100MVA):"; Ts "Sample time:"
      mask init:
      | Pnom_xfo=ParNom(1);
      | Freq=ParNom(2);
      | Bsec_pu100=100e6/Vsec_svc/Vsec_svc/3;
      | w=2*pi*Freq;
      | Bpu_TCR=-1/L_TCR/w/Bsec_pu100;
      | Bpu_TSC=1/(1/w/C_TSC-L_TSC*w)/Bsec_pu100;
      | B=1:-0.0025:0.0;
      | B=B';
      | for i=1:401,
      |       if B(i) <= 0,
      | 	ang = 0;
      |       elseif B(i) >= 1,
      | 	ang = pi;
      |       else,
      | 	a = pi; e = .0001;
      | 	da = a;
      | 	while abs(da)>e,
      | 		da = (pi*B(i)-a+sin(a))/(1-cos(a));
      | 		a = a + da;
      | 	end;
      | 	ang = a;
      |       end;
      |       A(i)=(180-ang*180/pi)/2+90;
      | end
      | A=A';
      | B=-B;
  Firing Unit : Subsystem  mask(Firing Unit){FiringMode=Synchronized, Nstep=0, ParInit=[0 60], Ts=Ts}
      mask prompts: FiringMode "Firing mode"; Nstep "Total delay (in number of time step)"; ParInit "Initial phase and frequency of input: [ Phase (degree)  Freq (Hz) ]"; Ts "Sample time:"
      mask init:
      | PhaseInit=ParInit(1);
      | FreqInit=ParInit(2);
      mask TypeOptions FiringMode: Synchronized | Continuous
  Logical Operator : Logic  Operator=OR
  Manual  Switch : ManualSwitch
  Measurement System : Subsystem  mask(SVC measurement system){Vnom=735e3, ParI=[735e3*0.9998 0 60], Ts=Ts}
      mask prompts: Vnom "Nominal voltage (volts rms ph-ph)"; ParI "Initial input: [ Mag (volts rms ph-ph)  Phase (degree) Freq (Hz) ]"; Ts "Sample time:"
      mask init:
      | Mag_Init=ParI(1)/Vnom;
      | Phase_Init=ParI(2);
      | Freq_Init=ParI(3);
  Mux2 : Mux  Inputs=[1 5]
  Sum : Sum  Inputs=|++  SaturateOnIntegerOverflow=on
  Timer : powerlib_extras/Control  Blocks/Timer  t="[ 0  0.121  0.121+eps ]*100"  e="[0  1  0 ]"
  Timer2 : powerlib_extras/Control  Blocks/Timer  t="[ 0  0.4  0.6 ]"  e=[1 1 1 ]
  Voltage Regulator : Subsystem
  TCR : Outport
  TSC1 : Outport  Port=2
  TSC2 : Outport  Port=3
  TSC3 : Outport  Port=4
  wires:
  Timer/1 -> Logical Operator/1
  Firing Unit/2(TSC1_Pulses) -> Demux/1
  Measurement System/1(Vmes) -> Voltage Regulator/1(Vmes)
  Constant1/1 -> Voltage Regulator/2(Bref)
  Mux2/1 -> TSC1/1
  Demux/2 -> Mux2/2
  Logical Operator/1 -> Mux2/1
  Demux/1 -> Logical Operator/2
  Voltage Regulator/1(Bsvc) -> Distribution Unit/1(Bsvc)
  Sum/1 -> Voltage Regulator/3(Vref)
  Constant/1 -> Sum/1
  Timer2/1 -> Sum/2
  Vabc_prim/1 -> Manual  Switch/1
  Manual  Switch/1 -> Measurement System/1(Vabc)
  3-phase signal generator/1(abc) -> Manual  Switch/2
  Firing Unit/1(TCR_Pulses) -> TCR/1
  Firing Unit/3(TSC2_Pulses) -> TSC2/1
  Firing Unit/4(TSC3_Pulses) -> TSC3/1
  Distribution Unit/1(Alpha) -> Firing Unit/2(Alpha)
  Distribution Unit/2(TSC1_On) -> Firing Unit/3(TSC1_On)
  Distribution Unit/3(TSC2_On) -> Firing Unit/4(TSC2_On)
  Distribution Unit/4(TSC3_On) -> Firing Unit/5(TSC3_On)
  Vabc_sec/1 -> Firing Unit/1(Vabc)

== system MATLABPSB_BASED_MODELING_AND_Sim/SS1/TCR ==
  note: Firing pulses
  note: TCR
  P : Inport  PortDimensions=6
  Demux : Demux  Outputs=6
  Lab : powerlib/Elements/Series RLC Branch  LConnTagsString=__new0  RConnTagsString=__new0  BranchType=RL  Resistance=Rtcr  Inductance=Ltcr  SetiL0=off  InitialCurrent=0  Capacitance=1.0  Setx0=off  InitialVoltage=0  Measurements=Branch current
  Lbc : powerlib/Elements/Series RLC Branch  LConnTagsString=__new0  RConnTagsString=__new0  BranchType=RL  Resistance=Rtcr  Inductance=Ltcr  SetiL0=off  InitialCurrent=0  Capacitance=1.0  Setx0=off  InitialVoltage=0  Measurements=None
  Lca : powerlib/Elements/Series RLC Branch  LConnTagsString=__new0  RConnTagsString=__new0  BranchType=RL  Resistance=Rtcr  Inductance=Ltcr  SetiL0=off  InitialCurrent=0  Capacitance=1.0  Setx0=off  InitialVoltage=0  Measurements=None
  ThAB+ : powerlib/Power Electronics/Thyristor  Ron=Ron  Lon=0  Vf=Vf  IC=0  Rs=Rsnub  Cs=Csnub  Measurements=off
      settings: AttributesFormatString=\n
  ThAB- : powerlib/Power Electronics/Thyristor  Ron=Ron  Lon=0  Vf=Vf  IC=0  Rs=inf  Cs=0  Measurements=off
      settings: AttributesFormatString=\n
  ThBC+ : powerlib/Power Electronics/Thyristor  Ron=Ron  Lon=0  Vf=Vf  IC=0  Rs=Rsnub  Cs=Csnub  Measurements=off
      settings: AttributesFormatString=\n
  ThBC- : powerlib/Power Electronics/Thyristor  Ron=Ron  Lon=0  Vf=Vf  IC=0  Rs=inf  Cs=0  Measurements=off
      settings: AttributesFormatString=\n
  ThCA+ : powerlib/Power Electronics/Thyristor  Ron=Ron  Lon=0  Vf=Vf  IC=0  Rs=Rsnub  Cs=Csnub  Measurements=off
      settings: AttributesFormatString=\n
  ThCA- : powerlib/Power Electronics/Thyristor  Ron=Ron  Lon=0  Vf=Vf  IC=0  Rs=inf  Cs=0  Measurements=off
      settings: AttributesFormatString=\n
  A : PMIOPort  Port=1  Side=Left
  B : PMIOPort  Port=2  Side=Left
  C : PMIOPort  Port=3  Side=Left
  wires:
  P/1 -> Demux/1
  Demux/1 -> [Ap]
  Demux/2 -> [Am]
  Demux/3 -> [Bp]
  Demux/4 -> [Bm]
  Demux/5 -> [Cp]
  [Cp] -> ThCA+/1
  [Cm] -> ThCA-/1
  Demux/6 -> [Cm]
  [Bm] -> ThBC-/1
  [Bp] -> ThBC+/1
  [Am] -> ThAB-/1
  [Ap] -> ThAB+/1
  connections:
  ThAB-/LConn1 -- ThAB+/RConn1 -- Lab/LConn1
  ThAB+/LConn1 -- ThAB-/RConn1 -- Lca/RConn1 -- A/RConn1
  ThBC-/LConn1 -- Lbc/LConn1 -- ThBC+/RConn1
  Lab/RConn1 -- ThBC-/RConn1 -- ThBC+/LConn1 -- B/RConn1
  Lca/LConn1 -- ThCA-/LConn1 -- ThCA+/RConn1
  Lbc/RConn1 -- ThCA-/RConn1 -- ThCA+/LConn1 -- C/RConn1

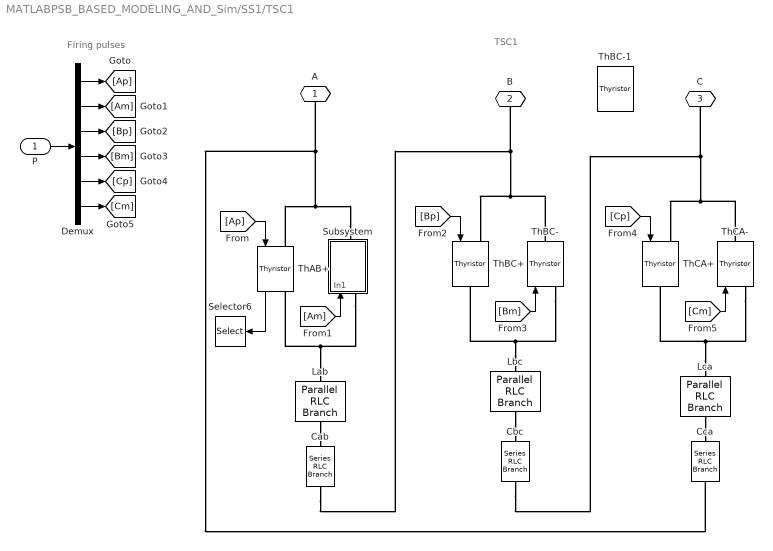
== system MATLABPSB_BASED_MODELING_AND_Sim/SS1/TSC1 ==
  note: Firing pulses
  note: TSC1
  P : Inport  PortDimensions=6
  Cab : powerlib/Elements/Series RLC Branch  LConnTagsString=__new0  RConnTagsString=__new0  BranchType=RC  Resistance=Rseries  Inductance=1.0  SetiL0=off  InitialCurrent=0  Capacitance=Ccmt  Setx0=off  InitialVoltage=0  Measurements=Branch voltage and current
  Cbc : powerlib/Elements/Series RLC Branch  LConnTagsString=__new0  RConnTagsString=__new0  BranchType=RC  Resistance=Rseries  Inductance=1.0  SetiL0=off  InitialCurrent=0  Capacitance=Ccmt  Setx0=off  InitialVoltage=0  Measurements=None
  Cca : powerlib/Elements/Series RLC Branch  LConnTagsString=__new0  RConnTagsString=__new0  BranchType=RC  Resistance=Rseries  Inductance=1.0  SetiL0=off  InitialCurrent=0  Capacitance=Ccmt  Setx0=off  InitialVoltage=0  Measurements=None
  Demux : Demux  Outputs=6
  Lab : powerlib/Elements/Parallel RLC Branch  LConnTagsString=a  RConnTagsString=__new0  BranchType=RL  Resistance=Rparallel  Inductance=Lcmt  SetiL0=off  InitialCurrent=0  Capacitance=1.0  Setx0=off  InitialVoltage=0  Measurements=None
  Lbc : powerlib/Elements/Parallel RLC Branch  LConnTagsString=a  RConnTagsString=__new0  BranchType=RL  Resistance=Rparallel  Inductance=Lcmt  SetiL0=off  InitialCurrent=0  Capacitance=1.0  Setx0=off  InitialVoltage=0  Measurements=None
  Lca : powerlib/Elements/Parallel RLC Branch  LConnTagsString=a  RConnTagsString=__new0  BranchType=RL  Resistance=Rparallel  Inductance=Lcmt  SetiL0=off  InitialCurrent=0  Capacitance=1.0  Setx0=off  InitialVoltage=0  Measurements=None
  Selector6 : Selector  InputPortWidth=2  IndexOptions=Index vector (dialog)  Indices=2  OutputSizes=1
  Subsystem : Subsystem  mask(Thyristor){Ron=Ron, Lon=0, Vf=Vf, IC=0, Rs=inf, Cs=0, Measurements=off}
      mask prompts: Ron "Resistance Ron (Ohms) :"; Lon "Inductance Lon (H) :"; Vf "Forward voltage Vf (V) :"; IC "Initial current Ic (A) :"; Rs "Snubber resistance Rs (Ohms) :"; Cs "Snubber capacitance Cs (F) :"; Measurements "Show measurement port"
      mask help:
      | Thyristor in parallel with a series RC snubber circuit.
      | In on-state the Thyristor model has an internal resistance (Ron) and inductance (Lon).
      | For most applications the internal inductance should be set to zero.
      | In off-state the Thyristor as an infinite impedance.
      mask Help: helpview(psbhelp);
      mask TypeOptions Ron: ThAB-/Ron
      mask TypeOptions Lon: ThAB-/Lon
      mask TypeOptions Vf: ThAB-/Vf
      mask TypeOptions IC: ThAB-/IC
      mask TypeOptions Rs: ThAB-/Rs
      mask TypeOptions Cs: ThAB-/Cs
      mask TypeOptions Measurements: ThAB-/Measurements
  ThAB+ : powerlib/Power Electronics/Thyristor  Ron=Ron  Lon=0  Vf=Vf  IC=0  Rs=Rsnub  Cs=Csnub  Measurements=on
      settings: AttributesFormatString=\n
  ThBC+ : powerlib/Power Electronics/Thyristor  Ron=Ron  Lon=0  Vf=Vf  IC=0  Rs=Rsnub  Cs=Csnub  Measurements=off
      settings: AttributesFormatString=\n
  ThBC- : powerlib/Power Electronics/Thyristor  Ron=Ron  Lon=0  Vf=Vf  IC=0  Rs=inf  Cs=0  Measurements=off
      settings: AttributesFormatString=\n
  ThBC-1 : powerlib/Power Electronics/Thyristor  Ron=Ron  Lon=0  Vf=Vf  IC=0  Rs=inf  Cs=0  Measurements=off
      settings: AttributesFormatString=\n
  ThCA+ : powerlib/Power Electronics/Thyristor  Ron=Ron  Lon=0  Vf=Vf  IC=0  Rs=Rsnub  Cs=Csnub  Measurements=off
      settings: AttributesFormatString=\n
  ThCA- : powerlib/Power Electronics/Thyristor  Ron=Ron  Lon=0  Vf=Vf  IC=0  Rs=inf  Cs=0  Measurements=off
      settings: AttributesFormatString=\n
  A : PMIOPort  Port=1  Side=Left
  B : PMIOPort  Port=2  Side=Left
  C : PMIOPort  Port=3  Side=Left
  wires:
  P/1 -> Demux/1
  [Ap] -> ThAB+/1
  Demux/1 -> [Ap]
  Demux/2 -> [Am]
  Demux/3 -> [Bp]
  Demux/4 -> [Bm]
  Demux/5 -> [Cp]
  [Am] -> Subsystem/1(In1)
  [Bp] -> ThBC+/1
  [Bm] -> ThBC-/1
  [Cp] -> ThCA+/1
  [Cm] -> ThCA-/1
  Demux/6 -> [Cm]
  ThAB+/1 -> Selector6/1
  connections:
  Lab/RConn1 -- Cab/LConn1
  Subsystem/LConn1 -- Lab/LConn1 -- ThAB+/RConn1
  Subsystem/RConn1 -- Cca/RConn1 -- A/RConn1 -- ThAB+/LConn1
  Lbc/LConn1 -- ThBC-/LConn1 -- ThBC+/RConn1
  Cab/RConn1 -- ThBC-/RConn1 -- ThBC+/LConn1 -- B/RConn1
  Lca/LConn1 -- ThCA-/LConn1 -- ThCA+/RConn1
  Cbc/RConn1 -- ThCA-/RConn1 -- ThCA+/LConn1 -- C/RConn1
  Lbc/RConn1 -- Cbc/LConn1
  Lca/RConn1 -- Cca/LConn1

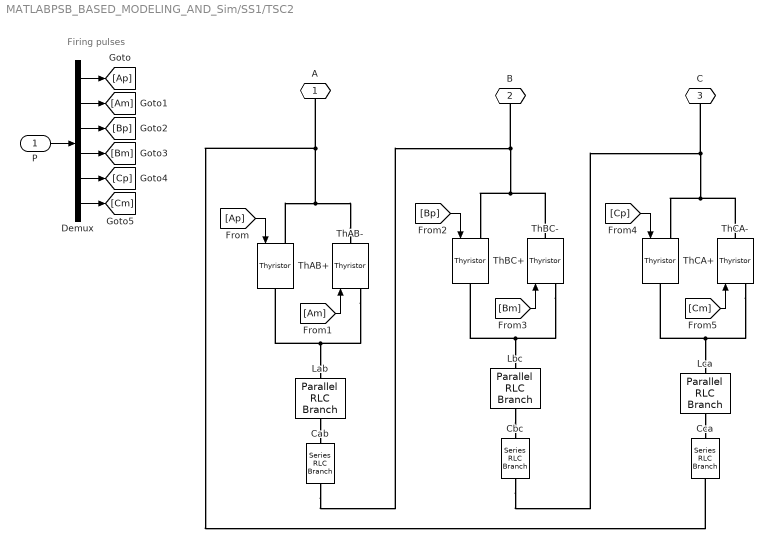
== system MATLABPSB_BASED_MODELING_AND_Sim/SS1/TSC2 ==
  note: Firing pulses
  P : Inport  PortDimensions=6
  Cab : powerlib/Elements/Series RLC Branch  LConnTagsString=__new0  RConnTagsString=__new0  BranchType=RC  Resistance=Rseries  Inductance=1.0  SetiL0=off  InitialCurrent=0  Capacitance=Ccmt  Setx0=off  InitialVoltage=0  Measurements=Branch voltage and current
  Cbc : powerlib/Elements/Series RLC Branch  LConnTagsString=__new0  RConnTagsString=__new0  BranchType=RC  Resistance=Rseries  Inductance=1.0  SetiL0=off  InitialCurrent=0  Capacitance=Ccmt  Setx0=off  InitialVoltage=0  Measurements=None
  Cca : powerlib/Elements/Series RLC Branch  LConnTagsString=__new0  RConnTagsString=__new0  BranchType=RC  Resistance=Rseries  Inductance=1.0  SetiL0=off  InitialCurrent=0  Capacitance=Ccmt  Setx0=off  InitialVoltage=0  Measurements=None
  Demux : Demux  Outputs=6
  Lab : powerlib/Elements/Parallel RLC Branch  LConnTagsString=a  RConnTagsString=__new0  BranchType=RL  Resistance=Rparallel  Inductance=Lcmt  SetiL0=off  InitialCurrent=0  Capacitance=1.0  Setx0=off  InitialVoltage=0  Measurements=None
  Lbc : powerlib/Elements/Parallel RLC Branch  LConnTagsString=a  RConnTagsString=__new0  BranchType=RL  Resistance=Rparallel  Inductance=Lcmt  SetiL0=off  InitialCurrent=0  Capacitance=1.0  Setx0=off  InitialVoltage=0  Measurements=None
  Lca : powerlib/Elements/Parallel RLC Branch  LConnTagsString=a  RConnTagsString=__new0  BranchType=RL  Resistance=Rparallel  Inductance=Lcmt  SetiL0=off  InitialCurrent=0  Capacitance=1.0  Setx0=off  InitialVoltage=0  Measurements=None
  ThAB+ : powerlib/Power Electronics/Thyristor  Ron=Ron  Lon=0  Vf=Vf  IC=0  Rs=Rsnub  Cs=Csnub  Measurements=off
      settings: AttributesFormatString=\n
  ThAB- : powerlib/Power Electronics/Thyristor  Ron=Ron  Lon=0  Vf=Vf  IC=0  Rs=inf  Cs=0  Measurements=off
      settings: AttributesFormatString=\n
  ThBC+ : powerlib/Power Electronics/Thyristor  Ron=Ron  Lon=0  Vf=Vf  IC=0  Rs=Rsnub  Cs=Csnub  Measurements=off
      settings: AttributesFormatString=\n
  ThBC- : powerlib/Power Electronics/Thyristor  Ron=Ron  Lon=0  Vf=Vf  IC=0  Rs=inf  Cs=0  Measurements=off
      settings: AttributesFormatString=\n
  ThCA+ : powerlib/Power Electronics/Thyristor  Ron=Ron  Lon=0  Vf=Vf  IC=0  Rs=Rsnub  Cs=Csnub  Measurements=off
      settings: AttributesFormatString=\n
  ThCA- : powerlib/Power Electronics/Thyristor  Ron=Ron  Lon=0  Vf=Vf  IC=0  Rs=inf  Cs=0  Measurements=off
      settings: AttributesFormatString=\n
  A : PMIOPort  Port=1  Side=Left
  B : PMIOPort  Port=2  Side=Left
  C : PMIOPort  Port=3  Side=Left
  wires:
  Demux/6 -> [Cm]
  [Cm] -> ThCA-/1
  [Cp] -> ThCA+/1
  [Bm] -> ThBC-/1
  [Bp] -> ThBC+/1
  [Am] -> ThAB-/1
  Demux/5 -> [Cp]
  Demux/4 -> [Bm]
  Demux/3 -> [Bp]
  Demux/2 -> [Am]
  Demux/1 -> [Ap]
  [Ap] -> ThAB+/1
  P/1 -> Demux/1
  connections:
  Lca/RConn1 -- Cca/LConn1
  Lbc/RConn1 -- Cbc/LConn1
  C/RConn1 -- ThCA+/LConn1 -- ThCA-/RConn1 -- Cbc/RConn1
  ThCA+/RConn1 -- ThCA-/LConn1 -- Lca/LConn1
  B/RConn1 -- ThBC+/LConn1 -- ThBC-/RConn1 -- Cab/RConn1
  ThBC+/RConn1 -- ThBC-/LConn1 -- Lbc/LConn1
  ThAB-/RConn1 -- ThAB+/LConn1 -- A/RConn1 -- Cca/RConn1
  ThAB+/RConn1 -- ThAB-/LConn1 -- Lab/LConn1
  Lab/RConn1 -- Cab/LConn1
